simulink model "text100"  (R2020b)
settings: Solver=VariableStepAuto  StartTime=0.0  StopTime=10.0  RelTol=1e-3
libraries: powerlib x16, eeDiscretePi x1, simulink x1, powerlib_extras x1
settings Model: Creator=38061  LastModifiedBy=38061

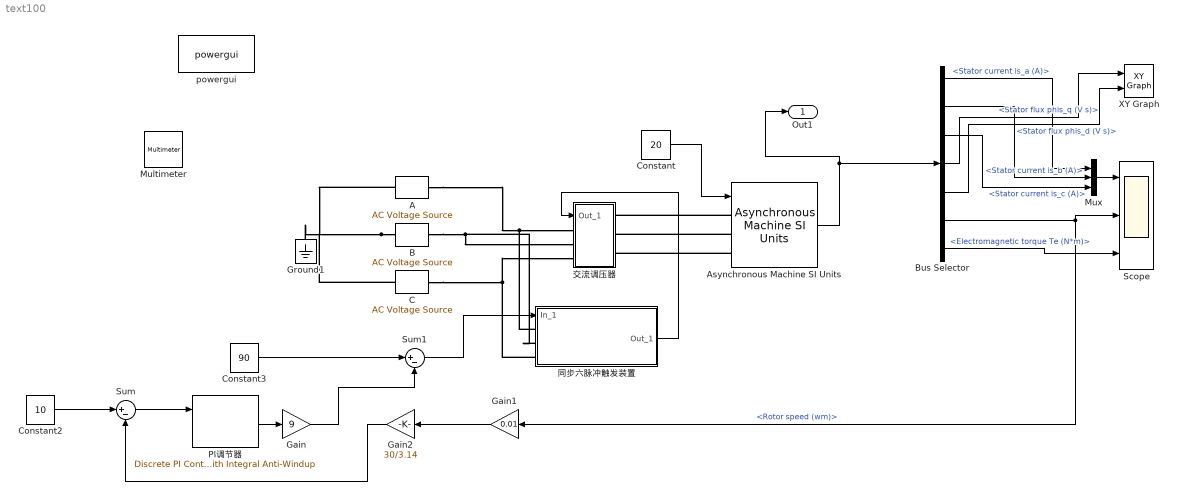
== system text100 ==
  A : powerlib/Electrical Sources/AC Voltage Source  Amplitude=220  Phase=0  Frequency=50  SampleTime=0  Measurements=None  BusType=swing  Pref=10e3  Qref=0  Qmin=-inf  Qmax=+inf
  Asynchronous Machine SI Units : powerlib/Machines/Asynchronous Machine SI Units  RotorType=Squirrel-cage  PresetModel=No  MechanicalLoad=Torque Tm  ShowDetailedParameters=on  ReferenceFrame=Rotor  Units=SI  MeasurementBus=off  NominalParameters=[1.845e+04 380 50]  Stator=[0.5968 0.0003495]  Rotor=[0.6258 0.005473]  Cage1=[0.4155 0.002066]  Cage2=[0.4168 0.0003495]  Lm=0.0354  Mechanical=[0.05 0.005879 2]  PolePairs=2  InitialConditions=[0 0 0 0 0 0 0 0]  SimulateSaturation=off  Saturation=[14.03593122, 27.81365428, 53.79336849, 72.68890987, 97.98006896, 148.6815601, 215.7428561, 302.9841135, 428.7778367 ; 230, 322, 414, 460, 506, 552, 598, 644, 690]  LoadFlowParameters=1492000  TsPowergui=0  TsBlock=-1  IterativeModel=Trapezoidal non iterative  IterativeDiscreteModel=Trapezoidal non iterative  Pmec=1.492e+006
  B : powerlib/Electrical Sources/AC Voltage Source  Amplitude=220  Phase=120  Frequency=50  SampleTime=0  Measurements=None  BusType=swing  Pref=10e3  Qref=0  Qmin=-inf  Qmax=+inf
  Bus Selector : BusSelector  OutputSignals=Stator measurements.Stator current is_a (A),Stator measurements.Stator current is_b (A),Stator measurements.Stator current is_c (A),Stator measurements.Stator flux phis_q (V s),Stator measurements.Stator flux phis_d (V s),Mechanical.Rotor speed (wm),Mechanical.Electromagnetic torque Te (N*m)
  C : powerlib/Electrical Sources/AC Voltage Source  Amplitude=220  Phase=240  Frequency=50  SampleTime=0  Measurements=None  BusType=swing  Pref=10e3  Qref=0  Qmin=-inf  Qmax=+inf
  Constant : Constant  Value=20
  Constant2 : Constant  Value=10
  Constant3 : Constant  Value=90
  Gain : Gain  Gain=9
  Gain1 : Gain  Gain=0.01
  Gain2 : Gain  Gain=30/3.14
  Ground1 : powerlib/Elements/Ground  LConnTagsString=a
  Multimeter : powerlib/Measurements/Multimeter  PhasorSimulation=off  OutputType=Complex  sel=1  L=1  Gain=0  yselected={}  PSBOutputType=1  PSBequivalent=0  AxesSetting=[0,0.1,-100,100]  Display=0  SavedBlockNames=-11
  Mux : Mux  Inputs=3
  PI调节器 : eeDiscretePi/Discrete PI Controller with Integral Anti-Windup  Kp=2  Ki=0.6  x0=0  B=10  A=-10  Ts=50e-6
      settings: SourceProductBaseCode=PS
  Scope : Scope  NumInputPorts=3
  Sum : Sum  Inputs=|+-
  Sum1 : Sum  Inputs=|+-
  XY Graph : simulink/Sinks/XY Graph  xmin=-2  xmax=2  ymin=-1  ymax=1  st=0.0001
  powergui : powerlib/powergui  Priority=1  SimulationMode=Continuous  SampleTime=50e-6  frequency=60  Iterations=50  frequencyindice=50  Pbase=100e6  ErrMax=1e-4  UnitsV=kV  UnitsW=MW  buscounter=0  FunctionMessages=off  echomessages=off  EnableUseOfTLC=off  CurrentSourceSwitches=off  DisableSnubberDevices=off  DisableRonSwitches=off  DisableVfSwitches=off  DisplayEquations=off  AutomaticDiscreteSolvers=off  SolverType=Tustin/Backward Euler (TBE)  Interpol=off  ExternalGateDelay=off  methode=off  Ts=100  x0status=blocks  SPID=on  SwTol=0  HookPort=off  NonlinearTolerance=1e-4  nMaxIteration=100  ContinueOnMaxIteration=off  RestoreLinks=warning  ResistiveCurrentMeasurement=off  Frange=[0:2:500]  Ylog=off  Xlog=on  ShowGrid=off  save=off  variable=ZData  structure=0  ZoomFFT=off  StartTime=0.0  cycles=1  DisplayStyle=1  fundamental=60  FreqAxis=off  MaxFrequency=1000  frequencyindicesteady=1  RmsSteady=1  display=off
  交流调压器 : Subsystem
  同步六脉冲触发装置 : Subsystem
  Out1 : Outport
  wires:
  Constant/1 -> Asynchronous Machine SI Units/1
  同步六脉冲触发装置/1(Out_1) -> 交流调压器/1(Out_1)
  Asynchronous Machine SI Units/1 -> Out1/1, Bus Selector/1
  Constant2/1 -> Sum/1
  PI调节器/1 -> Gain/1
  Gain2/1 -> Sum/2
  Sum/1 -> PI调节器/1
  Sum1/1 -> 同步六脉冲触发装置/1(In_1)
  Gain1/1 -> Gain2/1
  Constant3/1 -> Sum1/1
  Gain/1 -> Sum1/2
  Bus Selector/1 -> Mux/1  "<Stator current is_a (A)>"
  Bus Selector/2 -> Mux/2  "<Stator current is_b (A)>"
  Bus Selector/3 -> Mux/3  "<Stator current is_c (A)>"
  Mux/1 -> Scope/1
  Bus Selector/4 -> XY Graph/1  "<Stator flux phis_q (V s)>"
  Bus Selector/5 -> XY Graph/2  "<Stator flux phis_d (V s)>"
  Bus Selector/6 -> Scope/2, Gain1/1  "<Rotor speed (wm)>"
  Bus Selector/7 -> Scope/3  "<Electromagnetic torque Te (N*m)>"
  connections:
  B/LConn1 -- Ground1/LConn1 -- C/LConn1 -- A/LConn1
  A/RConn1 -- 同步六脉冲触发装置/LConn1 -- 交流调压器/LConn1
  B/RConn1 -- 同步六脉冲触发装置/LConn2 -- 交流调压器/LConn2
  C/RConn1 -- 同步六脉冲触发装置/LConn3 -- 交流调压器/LConn3
  Asynchronous Machine SI Units/LConn1 -- 交流调压器/RConn1
  Asynchronous Machine SI Units/LConn2 -- 交流调压器/RConn2
  Asynchronous Machine SI Units/LConn3 -- 交流调压器/RConn3

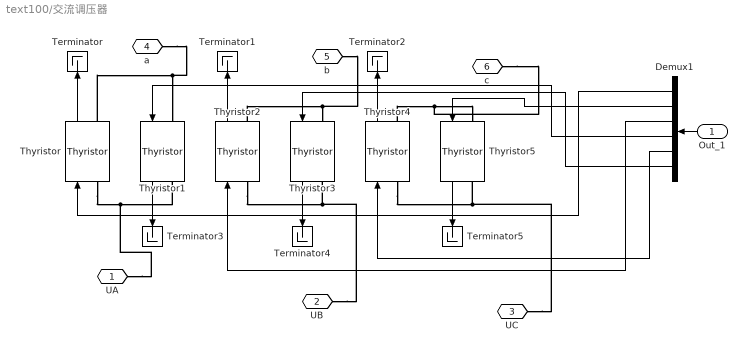
== system text100/交流调压器 ==
  Out_1 : Inport
  Demux1 : Demux  Outputs=6
  Terminator{,1..5} (6 alike) : Terminator
  Thyristor{,1..5} (6 alike) : powerlib/Power Electronics/Thyristor  Ron=0.001  Lon=0  Vf=0.8  IC=0  Rs=500  Cs=250e-9  Measurements=on
  UA : PMIOPort  Side=Left
  UB : PMIOPort  Port=2  Side=Left
  UC : PMIOPort  Port=3  Side=Left
  a : PMIOPort  Port=4  Side=Right
  b : PMIOPort  Port=5  Side=Right
  c : PMIOPort  Port=6  Side=Right
  wires:
  Thyristor1/1 -> Terminator3/1
  Thyristor3/1 -> Terminator4/1
  Demux1/1 -> Thyristor/1
  Thyristor2/1 -> Terminator1/1
  Thyristor4/1 -> Terminator2/1
  Thyristor/1 -> Terminator/1
  Thyristor5/1 -> Terminator5/1
  Demux1/3 -> Thyristor2/1
  Demux1/5 -> Thyristor4/1
  Demux1/2 -> Thyristor5/1
  Demux1/6 -> Thyristor3/1
  Demux1/4 -> Thyristor1/1
  Out_1/1 -> Demux1/1
  connections:
  Thyristor2/RConn1 -- b/RConn1 -- Thyristor3/LConn1
  Thyristor4/RConn1 -- c/RConn1 -- Thyristor5/LConn1
  Thyristor4/LConn1 -- UC/RConn1 -- Thyristor5/RConn1
  Thyristor/LConn1 -- UA/RConn1 -- Thyristor1/RConn1
  Thyristor2/LConn1 -- UB/RConn1 -- Thyristor3/RConn1
  Thyristor/RConn1 -- a/RConn1 -- Thyristor1/LConn1

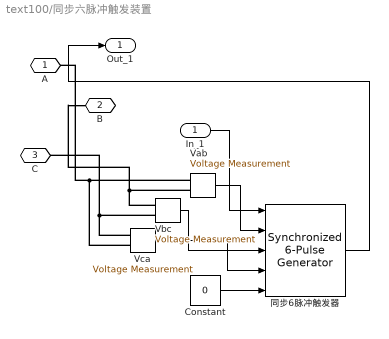
== system text100/同步六脉冲触发装置 ==
  In_1 : Inport
  Constant : Constant  Value=0
  Vab : powerlib/Measurements/Voltage Measurement  PhasorSimulation=off  OutputType=Complex  PSBequivalent=0
  Vbc : powerlib/Measurements/Voltage Measurement  PhasorSimulation=off  OutputType=Complex  PSBequivalent=0
  Vca : powerlib/Measurements/Voltage Measurement  PhasorSimulation=off  OutputType=Complex  PSBequivalent=0
  同步6脉冲触发器 : powerlib_extras/Control  Blocks/Synchronized 6-Pulse Generator  freq=50  pwidth=10  Double_Pulse=off
      settings: SourceProductBaseCode=PS
  A : PMIOPort  Side=Left
  B : PMIOPort  Port=2  Side=Left
  C : PMIOPort  Port=3  Side=Left
  Out_1 : Outport
  wires:
  同步6脉冲触发器/1 -> Out_1/1
  Vca/1 -> 同步6脉冲触发器/4
  Vab/1 -> 同步6脉冲触发器/2
  Constant/1 -> 同步6脉冲触发器/5
  Vbc/1 -> 同步6脉冲触发器/3
  In_1/1 -> 同步6脉冲触发器/1
  connections:
  Vca/LConn1 -- Vbc/LConn2 -- C/RConn1
  Vca/LConn2 -- Vab/LConn1 -- A/RConn1
  Vbc/LConn1 -- Vab/LConn2 -- B/RConn1
